simulink model "Roll_Autopilot"  (R2017b)
settings: Solver=VariableStepAuto  StartTime=0.0  StopTime=10.0  RelTol=1e-3
model workspace (MAT data in the model file):
  ContractValidatorBlocksMap = containers.Map
  ContractValidatorBlocksMap.serialization.keys = {'Roll_Autopilot/Roll_Autopilot_RollAutopilotSpec/validator', 'Roll_Autopilot/Roll_Autopilot_RollAutopilotSpec1/validator'}
  ContractValidatorBlocksMap.serialization.values{1}.block = 'Roll_Autopilot/Roll_Autopilot_RollAutopilotSpec/validator'
  ContractValidatorBlocksMap.serialization.values{1}.assumePorts = 0
  ContractValidatorBlocksMap.serialization.values{1}.guaranteePorts = 6
  ContractValidatorBlocksMap.serialization.values{1}.modeBlocksPorts = 2
  ContractValidatorBlocksMap.serialization.values{1}.portHandles.Inport = [3068.00048828 3069.00048828 3070.00048828 3071.00048828 3072.00231934 3074.00231934 3078.00231934 3079.00231934]
  ContractValidatorBlocksMap.serialization.values{1}.portHandles.Outport = 3080.00231934
  ContractValidatorBlocksMap.serialization.values{1}.portHandles.Enable = []
  ContractValidatorBlocksMap.serialization.values{1}.portHandles.Trigger = []
  ContractValidatorBlocksMap.serialization.values{1}.portHandles.State = []
  ContractValidatorBlocksMap.serialization.values{1}.portHandles.LConn = []
  ContractValidatorBlocksMap.serialization.values{1}.portHandles.RConn = []
  ContractValidatorBlocksMap.serialization.values{1}.portHandles.Ifaction = []
  ContractValidatorBlocksMap.serialization.values{1}.portHandles.Reset = []
  ContractValidatorBlocksMap.serialization.values{1}.portConnectivity(1).Type = '1'
  ContractValidatorBlocksMap.serialization.values{1}.portConnectivity(1).Position = [31840 -150]
  ContractValidatorBlocksMap.serialization.values{1}.portConnectivity(1).SrcBlock = 1525.00219727
  ContractValidatorBlocksMap.serialization.values{1}.portConnectivity(1).SrcPort = 0
  ContractValidatorBlocksMap.serialization.values{1}.portConnectivity(1).DstBlock = []
  ContractValidatorBlocksMap.serialization.values{1}.portConnectivity(1).DstPort = []
  ContractValidatorBlocksMap.serialization.values{1}.portConnectivity(2).Type = '2'
  ContractValidatorBlocksMap.serialization.values{1}.portConnectivity(2).Position = [31840 -85]
  ContractValidatorBlocksMap.serialization.values{1}.portConnectivity(2).SrcBlock = 1545.00048828
  ContractValidatorBlocksMap.serialization.values{1}.portConnectivity(2).SrcPort = 0
  ContractValidatorBlocksMap.serialization.values{1}.portConnectivity(2).DstBlock = []
  ContractValidatorBlocksMap.serialization.values{1}.portConnectivity(2).DstPort = []
  ContractValidatorBlocksMap.serialization.values{1}.portConnectivity(3).Type = '3'
  ContractValidatorBlocksMap.serialization.values{1}.portConnectivity(3).Position = [31840 -20]
  ContractValidatorBlocksMap.serialization.values{1}.portConnectivity(3).SrcBlock = 1541.00048828
  ContractValidatorBlocksMap.serialization.values{1}.portConnectivity(3).SrcPort = 0
  ContractValidatorBlocksMap.serialization.values{1}.portConnectivity(3).DstBlock = []
  ContractValidatorBlocksMap.serialization.values{1}.portConnectivity(3).DstPort = []
  ContractValidatorBlocksMap.serialization.values{1}.portConnectivity(4).Type = '4'
  ContractValidatorBlocksMap.serialization.values{1}.portConnectivity(4).Position = [31840 45]
  ContractValidatorBlocksMap.serialization.values{1}.portConnectivity(4).SrcBlock = 1537.00048828
  ContractValidatorBlocksMap.serialization.values{1}.portConnectivity(4).SrcPort = 0
  ContractValidatorBlocksMap.serialization.values{1}.portConnectivity(4).DstBlock = []
  ContractValidatorBlocksMap.serialization.values{1}.portConnectivity(4).DstPort = []
  ContractValidatorBlocksMap.serialization.values{1}.portConnectivity(5).Type = '5'
  ContractValidatorBlocksMap.serialization.values{1}.portConnectivity(5).Position = [31840 110]
  ContractValidatorBlocksMap.serialization.values{1}.portConnectivity(5).SrcBlock = 1533.00219727
  ContractValidatorBlocksMap.serialization.values{1}.portConnectivity(5).SrcPort = 0
  ContractValidatorBlocksMap.serialization.values{1}.portConnectivity(5).DstBlock = []
  ContractValidatorBlocksMap.serialization.values{1}.portConnectivity(5).DstPort = []
  ContractValidatorBlocksMap.serialization.values{1}.portConnectivity(6).Type = '6'
  ContractValidatorBlocksMap.serialization.values{1}.portConnectivity(6).Position = [31840 175]
  ContractValidatorBlocksMap.serialization.values{1}.portConnectivity(6).SrcBlock = 1549.00048828
  ContractValidatorBlocksMap.serialization.values{1}.portConnectivity(6).SrcPort = 0
  ContractValidatorBlocksMap.serialization.values{1}.portConnectivity(6).DstBlock = []
  ContractValidatorBlocksMap.serialization.values{1}.portConnectivity(6).DstPort = []
  ContractValidatorBlocksMap.serialization.values{1}.portConnectivity(7).Type = '7'
  ContractValidatorBlocksMap.serialization.values{1}.portConnectivity(7).Position = [31840 240]
  ContractValidatorBlocksMap.serialization.values{1}.portConnectivity(7).SrcBlock = 2047.00048828
  ContractValidatorBlocksMap.serialization.values{1}.portConnectivity(7).SrcPort = 0
  ContractValidatorBlocksMap.serialization.values{1}.portConnectivity(7).DstBlock = []
  ContractValidatorBlocksMap.serialization.values{1}.portConnectivity(7).DstPort = []
  ContractValidatorBlocksMap.serialization.values{1}.portConnectivity(8).Type = '8'
  ContractValidatorBlocksMap.serialization.values{1}.portConnectivity(8).Position = [31840 305]
  ContractValidatorBlocksMap.serialization.values{1}.portConnectivity(8).SrcBlock = 2007.00048828
  ContractValidatorBlocksMap.serialization.values{1}.portConnectivity(8).SrcPort = 0
  ContractValidatorBlocksMap.serialization.values{1}.portConnectivity(8).DstBlock = []
  ContractValidatorBlocksMap.serialization.values{1}.portConnectivity(8).DstPort = []
  ContractValidatorBlocksMap.serialization.values{1}.portConnectivity(9).Type = '1'
  ContractValidatorBlocksMap.serialization.values{1}.portConnectivity(9).Position = [31975 80]
  ContractValidatorBlocksMap.serialization.values{1}.portConnectivity(9).SrcBlock = []
  ContractValidatorBlocksMap.serialization.values{1}.portConnectivity(9).SrcPort = []
  ContractValidatorBlocksMap.serialization.values{1}.portConnectivity(9).DstBlock = 2349.00292969
  ContractValidatorBlocksMap.serialization.values{1}.portConnectivity(9).DstPort = 0
  ContractValidatorBlocksMap.serialization.values{2}.block = 'Roll_Autopilot/Roll_Autopilot_RollAutopilotSpec1/validator'
  ContractValidatorBlocksMap.serialization.values{2}.assumePorts = 0
  ContractValidatorBlocksMap.serialization.values{2}.guaranteePorts = 6
  ContractValidatorBlocksMap.serialization.values{2}.modeBlocksPorts = 2
  ContractValidatorBlocksMap.serialization.values{2}.portHandles.Inport = [7302.00048828 7304.00048828 7306.00048828 7308.00048828 7313.00048828 7319.00048828 7322.00048828 7326.00048828]
  ContractValidatorBlocksMap.serialization.values{2}.portHandles.Outport = 7710.00048828
  ContractValidatorBlocksMap.serialization.values{2}.portHandles.Enable = []
  ContractValidatorBlocksMap.serialization.values{2}.portHandles.Trigger = []
  ContractValidatorBlocksMap.serialization.values{2}.portHandles.State = []
  ContractValidatorBlocksMap.serialization.values{2}.portHandles.LConn = []
  ContractValidatorBlocksMap.serialization.values{2}.portHandles.RConn = []
  ContractValidatorBlocksMap.serialization.values{2}.portHandles.Ifaction = []
  ContractValidatorBlocksMap.serialization.values{2}.portHandles.Reset = []
  ContractValidatorBlocksMap.serialization.values{2}.portConnectivity(1).Type = '1'
  ContractValidatorBlocksMap.serialization.values{2}.portConnectivity(1).Position = [74140 -150]
  ContractValidatorBlocksMap.serialization.values{2}.portConnectivity(1).SrcBlock = 3094.00231934
  ContractValidatorBlocksMap.serialization.values{2}.portConnectivity(1).SrcPort = 0
  ContractValidatorBlocksMap.serialization.values{2}.portConnectivity(1).DstBlock = []
  ContractValidatorBlocksMap.serialization.values{2}.portConnectivity(1).DstPort = []
  ContractValidatorBlocksMap.serialization.values{2}.portConnectivity(2).Type = '2'
  ContractValidatorBlocksMap.serialization.values{2}.portConnectivity(2).Position = [74140 -85]
  ContractValidatorBlocksMap.serialization.values{2}.portConnectivity(2).SrcBlock = 3118.00231934
  ContractValidatorBlocksMap.serialization.values{2}.portConnectivity(2).SrcPort = 0
  ContractValidatorBlocksMap.serialization.values{2}.portConnectivity(2).DstBlock = []
  ContractValidatorBlocksMap.serialization.values{2}.portConnectivity(2).DstPort = []
  ContractValidatorBlocksMap.serialization.values{2}.portConnectivity(3).Type = '3'
  ContractValidatorBlocksMap.serialization.values{2}.portConnectivity(3).Position = [74140 -20]
  ContractValidatorBlocksMap.serialization.values{2}.portConnectivity(3).SrcBlock = 3110.00231934
  ContractValidatorBlocksMap.serialization.values{2}.portConnectivity(3).SrcPort = 0
  ContractValidatorBlocksMap.serialization.values{2}.portConnectivity(3).DstBlock = []
  ContractValidatorBlocksMap.serialization.values{2}.portConnectivity(3).DstPort = []
  ContractValidatorBlocksMap.serialization.values{2}.portConnectivity(4).Type = '4'
  ContractValidatorBlocksMap.serialization.values{2}.portConnectivity(4).Position = [74140 45]
  ContractValidatorBlocksMap.serialization.values{2}.portConnectivity(4).SrcBlock = 3106.00231934
  ContractValidatorBlocksMap.serialization.values{2}.portConnectivity(4).SrcPort = 0
  ContractValidatorBlocksMap.serialization.values{2}.portConnectivity(4).DstBlock = []
  ContractValidatorBlocksMap.serialization.values{2}.portConnectivity(4).DstPort = []
  ContractValidatorBlocksMap.serialization.values{2}.portConnectivity(5).Type = '5'
  ContractValidatorBlocksMap.serialization.values{2}.portConnectivity(5).Position = [74140 110]
  ContractValidatorBlocksMap.serialization.values{2}.portConnectivity(5).SrcBlock = 3098.00231934
  ContractValidatorBlocksMap.serialization.values{2}.portConnectivity(5).SrcPort = 0
  ContractValidatorBlocksMap.serialization.values{2}.portConnectivity(5).DstBlock = []
  ContractValidatorBlocksMap.serialization.values{2}.portConnectivity(5).DstPort = []
  ContractValidatorBlocksMap.serialization.values{2}.portConnectivity(6).Type = '6'
  ContractValidatorBlocksMap.serialization.values{2}.portConnectivity(6).Position = [74140 175]
  ContractValidatorBlocksMap.serialization.values{2}.portConnectivity(6).SrcBlock = 3122.00231934
  ContractValidatorBlocksMap.serialization.values{2}.portConnectivity(6).SrcPort = 0
  ContractValidatorBlocksMap.serialization.values{2}.portConnectivity(6).DstBlock = []
  ContractValidatorBlocksMap.serialization.values{2}.portConnectivity(6).DstPort = []
  ContractValidatorBlocksMap.serialization.values{2}.portConnectivity(7).Type = '7'
  ContractValidatorBlocksMap.serialization.values{2}.portConnectivity(7).Position = [74140 240]
  ContractValidatorBlocksMap.serialization.values{2}.portConnectivity(7).SrcBlock = 3628.00061035
  ContractValidatorBlocksMap.serialization.values{2}.portConnectivity(7).SrcPort = 0
  ContractValidatorBlocksMap.serialization.values{2}.portConnectivity(7).DstBlock = []
  ContractValidatorBlocksMap.serialization.values{2}.portConnectivity(7).DstPort = []
  ContractValidatorBlocksMap.serialization.values{2}.portConnectivity(8).Type = '8'
  ContractValidatorBlocksMap.serialization.values{2}.portConnectivity(8).Position = [74140 305]
  ContractValidatorBlocksMap.serialization.values{2}.portConnectivity(8).SrcBlock = 3594.00061035
  ContractValidatorBlocksMap.serialization.values{2}.portConnectivity(8).SrcPort = 0
  ContractValidatorBlocksMap.serialization.values{2}.portConnectivity(8).DstBlock = []
  ContractValidatorBlocksMap.serialization.values{2}.portConnectivity(8).DstPort = []
  ContractValidatorBlocksMap.serialization.values{2}.portConnectivity(9).Type = '1'
  ContractValidatorBlocksMap.serialization.values{2}.portConnectivity(9).Position = [74275 80]
  ContractValidatorBlocksMap.serialization.values{2}.portConnectivity(9).SrcBlock = []
  ContractValidatorBlocksMap.serialization.values{2}.portConnectivity(9).SrcPort = []
  ContractValidatorBlocksMap.serialization.values{2}.portConnectivity(9).DstBlock = 4161.00061035
  ContractValidatorBlocksMap.serialization.values{2}.portConnectivity(9).DstPort = 0
  ContractValidatorBlocksMap.serialization.uniformity = 0
  ContractValidatorBlocksMap.serialization.keyType = 'char'
  ContractValidatorBlocksMap.serialization.valueType = 'any'
undefined symbols (not defined in the file): contractAfterSimulation, contractBeforeSimulation, ContractBlock, ContractEnsureBlock, ContractGuaranteeBlock, ContractModeBlock, ContractRequireBlock, ContractValidatorBlock, saveValidatorParameters, Ts
libraries: cocosimLibs x20, simulink x2
(part 1 of 2)
settings Model: Creator=hbourbou  LastModifiedBy=hbourbou
settings DataIOCC: ReturnWorkspaceOutputs=on
settings SFSimCC: SimUseLocalCustomCode=on
settings RTWCC: RTWUseLocalCustomCode=on

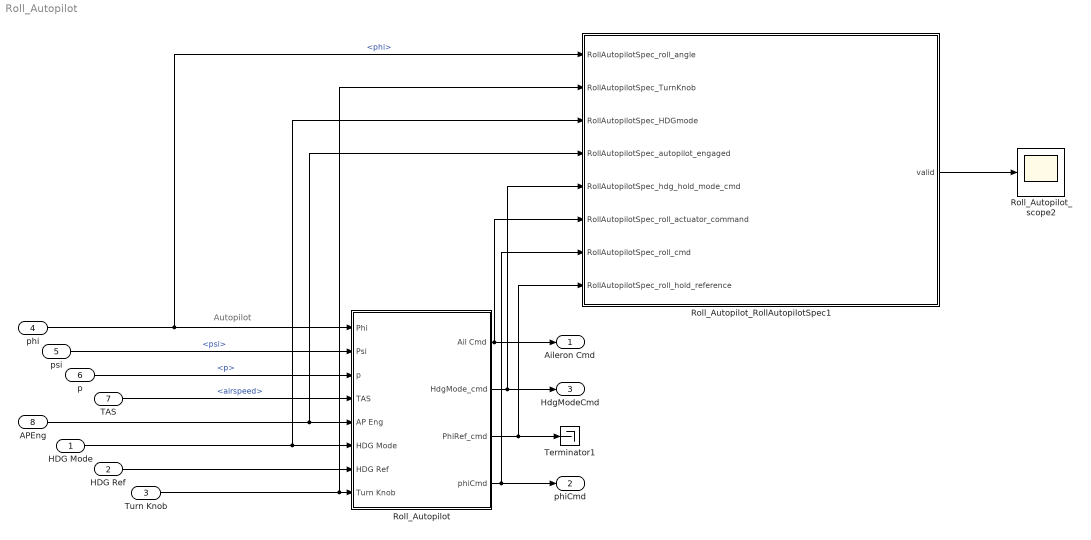
== system Roll_Autopilot ==
  note: Autopilot
  HDG Mode : Inport  OutMin=0  OutMax=1  OutDataTypeStr=boolean  PortDimensions=1
  HDG Ref : Inport  Port=2  OutMin=-180  OutMax=180  OutDataTypeStr=double  PortDimensions=1
  Turn Knob : Inport  Port=3  OutMin=-45  OutMax=45  OutDataTypeStr=double  PortDimensions=1
  phi : Inport  Port=4
  psi : Inport  Port=5
  p : Inport  Port=6
  TAS : Inport  Port=7
  APEng : Inport  Port=8  OutDataTypeStr=boolean
  Roll_Autopilot : Subsystem
  Roll_Autopilot_RollAutopilotSpec1 : Subsystem  mask(ContractBlock){ContractBlockType=ContractBlock}
      mask init:
      | set_param(gcb, 'LinkStatus', 'none');
      mask DialogControl DescTextVar Prompt: Contract block
      mask Display:
      | text(0.5, 0.5, '{\bf\fontsize{20}Contract}', 'hor', 'center', 'texmode','on');
      | blocks = find_system(gcb, 'LookUnderMasks','all', 'SearchDepth',1,'BlockType','Inport');
      | for i = 1 : length(blocks)
      |     blockName = get_param(blocks(i), 'Name');
      |     [path, blockName] = fileparts(char(blockName));
      |     port_label('input', i, blockName);
      | end
      | 
      | blocks = find_system(gcb, 'LookUnderMasks','all', 'SearchDepth',1,'BlockType','Outport');
      | for i = 1 : length(blocks)
      |     blockName = get_param(blocks(i), 'Name');
      |     [path, blockName] = fileparts(char(blockName));
      |     port_label('output', i, blockName);
      | end
  Roll_Autopilot_scope2 : Scope
  Terminator1 : Terminator
  Aileron Cmd : Outport  OutDataTypeStr=double  PortDimensions=1  SampleTime=[0.025000000000000001,0]  VectorParamsAs1DForOutWhenUnconnected=off
  phiCmd : Outport  Port=2  VectorParamsAs1DForOutWhenUnconnected=off
  HdgModeCmd : Outport  Port=3  VectorParamsAs1DForOutWhenUnconnected=off
  wires:
  APEng/1 -> Roll_Autopilot_RollAutopilotSpec1/4(RollAutopilotSpec_autopilot_engaged), Roll_Autopilot/5(AP Eng)
  TAS/1 -> Roll_Autopilot/4(TAS)  "<airspeed>"
  Roll_Autopilot/2(HdgMode_cmd) -> Roll_Autopilot_RollAutopilotSpec1/5(RollAutopilotSpec_hdg_hold_mode_cmd), HdgModeCmd/1
  Turn Knob/1 -> Roll_Autopilot_RollAutopilotSpec1/2(RollAutopilotSpec_TurnKnob), Roll_Autopilot/8(Turn Knob)
  phi/1 -> Roll_Autopilot_RollAutopilotSpec1/1(RollAutopilotSpec_roll_angle), Roll_Autopilot/1(Phi)  "<phi>"
  HDG Mode/1 -> Roll_Autopilot_RollAutopilotSpec1/3(RollAutopilotSpec_HDGmode), Roll_Autopilot/6(HDG Mode)
  HDG Ref/1 -> Roll_Autopilot/7(HDG Ref)
  p/1 -> Roll_Autopilot/3(p)  "<p>"
  Roll_Autopilot/1(Ail Cmd) -> Roll_Autopilot_RollAutopilotSpec1/6(RollAutopilotSpec_roll_actuator_command), Aileron Cmd/1
  psi/1 -> Roll_Autopilot/2(Psi)  "<psi>"
  Roll_Autopilot/4(phiCmd) -> Roll_Autopilot_RollAutopilotSpec1/7(RollAutopilotSpec_roll_cmd), phiCmd/1
  Roll_Autopilot/3(PhiRef_cmd) -> Roll_Autopilot_RollAutopilotSpec1/8(RollAutopilotSpec_roll_hold_reference), Terminator1/1
  Roll_Autopilot_RollAutopilotSpec1/1(valid) -> Roll_Autopilot_scope2/1

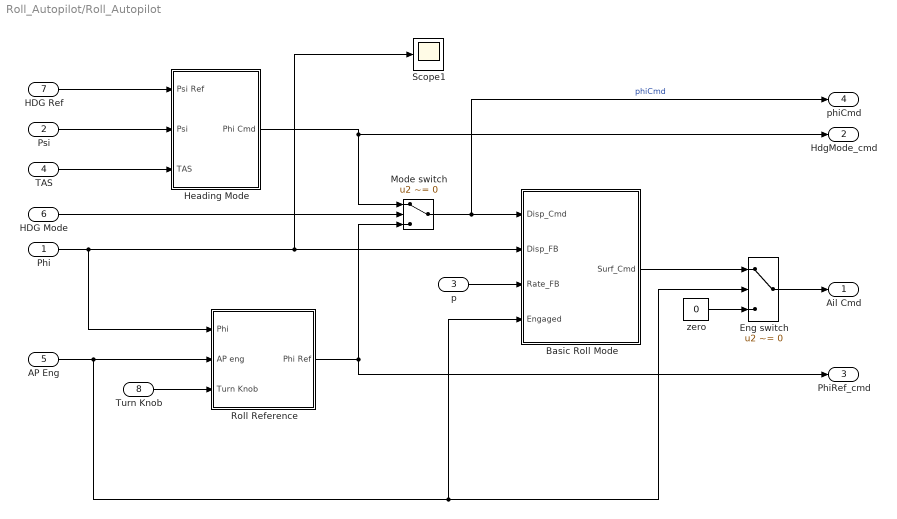
== system Roll_Autopilot/Roll_Autopilot ==
  Phi : Inport  OutMin=-180  OutMax=180  OutDataTypeStr=double  PortDimensions=1  SampleTime=1/40  Interpolate=off
  Psi : Inport  Port=2  OutMin=-180  OutMax=180  OutDataTypeStr=double  PortDimensions=1  SampleTime=1/40  Interpolate=off
  p : Inport  Port=3  OutMin=-180  OutMax=180  OutDataTypeStr=double  PortDimensions=1  Interpolate=off
  TAS : Inport  Port=4  OutMin=0  OutMax=1000  OutDataTypeStr=double  PortDimensions=1  SampleTime=1/40  Interpolate=off
  AP Eng : Inport  Port=5  OutDataTypeStr=boolean  PortDimensions=1  SampleTime=1/40  Interpolate=off
  HDG Mode : Inport  Port=6  OutDataTypeStr=boolean  PortDimensions=1  SampleTime=1/40  Interpolate=off
  HDG Ref : Inport  Port=7  OutMin=-180  OutMax=180  OutDataTypeStr=double  PortDimensions=1  SampleTime=1/40  Interpolate=off
  Turn Knob : Inport  Port=8  OutMin=-45  OutMax=45  OutDataTypeStr=double  PortDimensions=1  SampleTime=1/40  Interpolate=off
  Basic Roll Mode : Subsystem
  Eng switch : Switch  Criteria=u2 ~= 0
  Heading Mode : Subsystem
  Mode switch : Switch  Criteria=u2 ~= 0
  Roll Reference : Subsystem  TreatAsAtomicUnit=on
      settings: RTWSystemCode=Inline
  Scope1 : Scope
  zero : Constant  Value=0  OutDataTypeStr=double
  Ail Cmd : Outport  OutDataTypeStr=double  PortDimensions=1  SampleTime=1/40  VectorParamsAs1DForOutWhenUnconnected=off
  HdgMode_cmd : Outport  Port=2  VectorParamsAs1DForOutWhenUnconnected=off
  PhiRef_cmd : Outport  Port=3  VectorParamsAs1DForOutWhenUnconnected=off
  phiCmd : Outport  Port=4  VectorParamsAs1DForOutWhenUnconnected=off
  wires:
  HDG Ref/1 -> Heading Mode/1(Psi Ref)
  Heading Mode/1(Phi Cmd) -> HdgMode_cmd/1, Mode switch/1
  Mode switch/1 -> phiCmd/1, Basic Roll Mode/1(Disp_Cmd)  "phiCmd"
  Eng switch/1 -> Ail Cmd/1
  AP Eng/1 -> Roll Reference/2(AP eng), Basic Roll Mode/4(Engaged), Eng switch/2
  TAS/1 -> Heading Mode/3(TAS)
  HDG Mode/1 -> Mode switch/2
  Roll Reference/1(Phi Ref) -> Mode switch/3, PhiRef_cmd/1
  Turn Knob/1 -> Roll Reference/3(Turn Knob)
  zero/1 -> Eng switch/3
  p/1 -> Basic Roll Mode/3(Rate_FB)
  Phi/1 -> Scope1/1, Basic Roll Mode/2("Disp_FB "), Roll Reference/1(Phi)
  Psi/1 -> Heading Mode/2(Psi)
  Basic Roll Mode/1(Surf_Cmd) -> Eng switch/1

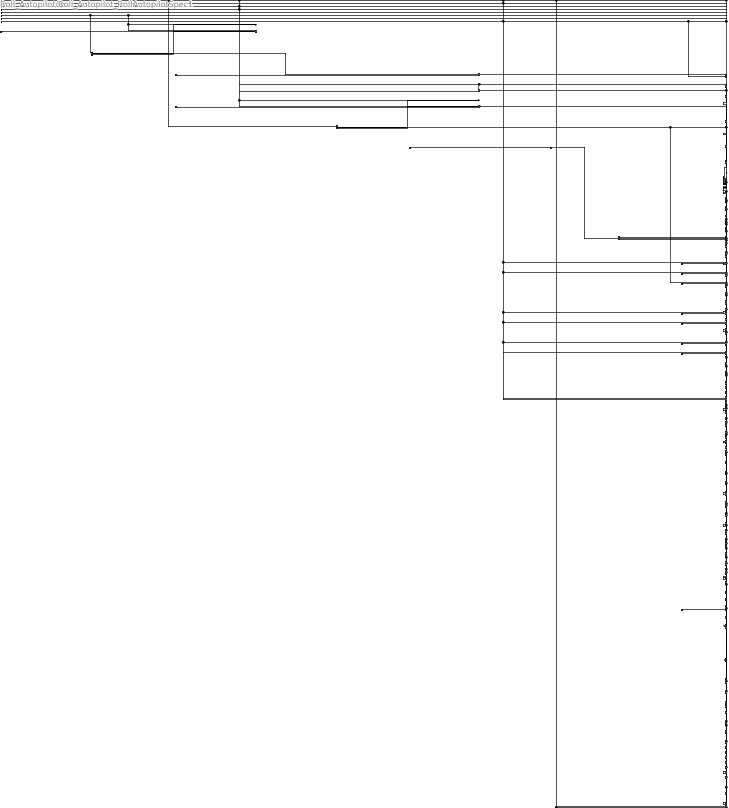
== system Roll_Autopilot/Roll_Autopilot_RollAutopilotSpec1 ==
  RollAutopilotSpec_roll_angle : Inport  OutDataTypeStr=double
  RollAutopilotSpec_TurnKnob : Inport  Port=2  OutDataTypeStr=double
  RollAutopilotSpec_HDGmode : Inport  Port=3  OutDataTypeStr=boolean
  RollAutopilotSpec_autopilot_engaged : Inport  Port=4  OutDataTypeStr=boolean
  RollAutopilotSpec_hdg_hold_mode_cmd : Inport  Port=5  OutDataTypeStr=double
  RollAutopilotSpec_roll_actuator_command : Inport  Port=6  OutDataTypeStr=double
  RollAutopilotSpec_roll_cmd : Inport  Port=7  OutDataTypeStr=double
  RollAutopilotSpec_roll_hold_reference : Inport  Port=8  OutDataTypeStr=double
  AP-001 : Subsystem  mask(ContractGuaranteeBlock){ContractBlockType=ContractGuaranteeBlock}
      mask init:
      | set_param(gcb, 'LinkStatus', 'none');
      mask DialogControl DescTextVar Prompt: Guarantee block
  AP-003A : Subsystem  mask(ContractGuaranteeBlock){ContractBlockType=ContractGuaranteeBlock}
      mask init:
      | set_param(gcb, 'LinkStatus', 'none');
      mask DialogControl DescTextVar Prompt: Guarantee block
  AP-003B : Subsystem  mask(ContractGuaranteeBlock){ContractBlockType=ContractGuaranteeBlock}
      mask init:
      | set_param(gcb, 'LinkStatus', 'none');
      mask DialogControl DescTextVar Prompt: Guarantee block
  AP-003C : Subsystem  mask(ContractGuaranteeBlock){ContractBlockType=ContractGuaranteeBlock}
      mask init:
      | set_param(gcb, 'LinkStatus', 'none');
      mask DialogControl DescTextVar Prompt: Guarantee block
  AP-003D : Subsystem  mask(ContractGuaranteeBlock){ContractBlockType=ContractGuaranteeBlock}
      mask init:
      | set_param(gcb, 'LinkStatus', 'none');
      mask DialogControl DescTextVar Prompt: Guarantee block
  AP-007 : Subsystem  mask(ContractGuaranteeBlock){ContractBlockType=ContractGuaranteeBlock}
      mask init:
      | set_param(gcb, 'LinkStatus', 'none');
      mask DialogControl DescTextVar Prompt: Guarantee block
  Arrow_xxRollAutopilotSpec_162_ni_7 : Delay  DelayLength=1  InitialCondition=1
  Arrow_xxRollAutopilotSpec_163_ni_9 : Delay  DelayLength=1  InitialCondition=1
  Arrow_xxRollAutopilotSpec_164_ni_12 : Delay  DelayLength=1  InitialCondition=1
  Arrow_xxRollAutopilotSpec_165_ni_16 : Delay  DelayLength=1  InitialCondition=1
  Arrow_xxRollAutopilotSpec_183_ni_3 : Delay  DelayLength=1  InitialCondition=1
  Ca_operator : Logic  Operator=NOT  AllPortsSameDT=off  OutDataTypeStr=boolean
  Cb_operator : Logic  AllPortsSameDT=off  OutDataTypeStr=boolean
  Cc_operator : RelationalOperator  OutDataTypeStr=boolean  RndMeth=Simplest
  Cc_rhs_2 : Constant  Value=30.0  OutDataTypeStr=double
  Cd_operator : Logic  AllPortsSameDT=off  OutDataTypeStr=boolean
  H_call : Subsystem
  H_call1 : Subsystem
  H_call11 : Subsystem
  PRE_xxRollAutopilotSpec_{8,13,17,22,33,38,42,44,59,64,68,73,84,89,93,95,109,114,118,123,133,138,142,144,184,187} (26 alike) : Delay  DelayLength=1  InitialCondition=0
  SI_call : Subsystem
  SI_call1 : Subsystem
  SI_call11 : Subsystem
  SI_call111 : Subsystem
  SI_call1111 : Subsystem
  SI_call11111 : Subsystem
  SI_call111111 : Subsystem
  SI_call1111111 : Subsystem
  SI_call11111111 : Subsystem
  branch_10_IF : Switch  Criteria=u2 ~= 0
  branch_11_IF : Switch  Criteria=u2 ~= 0
  branch_12_IF : Switch  Criteria=u2 ~= 0
  branch_13_IF : Switch  Criteria=u2 ~= 0
  branch_14_IF : Switch  Criteria=u2 ~= 0
  branch_15_IF : Switch  Criteria=u2 ~= 0
  branch_16_IF : Switch  Criteria=u2 ~= 0
  branch_8_IF : Switch  Criteria=u2 ~= 0
  branch_9_IF : Switch  Criteria=u2 ~= 0
  hdg_hold_mode : Subsystem  mask(ContractModeBlock){ContractBlockType=ContractModeBlock}
      mask init:
      | set_param(gcb, 'LinkStatus', 'none');
      mask DialogControl DescTextVar Prompt: Mode block
  hdg_hold_mode_ensure : Subsystem  mask(ContractEnsureBlock){ContractBlockType=ContractEnsureBlock}
      mask init:
      | set_param(gcb, 'LinkStatus', 'none');
      mask DialogControl DescTextVar Prompt: Ensure block
  hdg_hold_mode_ensure_cond : Logic  Inputs=1  AllPortsSameDT=off  OutDataTypeStr=boolean
  hdg_hold_mode_require : Subsystem  mask(ContractRequireBlock){ContractBlockType=ContractRequireBlock}
      mask init:
      | set_param(gcb, 'LinkStatus', 'none');
      mask DialogControl DescTextVar Prompt: Require block
  hdg_hold_mode_require_cond : Logic  Inputs=1  AllPortsSameDT=off  OutDataTypeStr=boolean
  no_other_lateral_mode_operator : Logic  Operator=NOT  AllPortsSameDT=off  OutDataTypeStr=boolean
  roll_hold_mode : Subsystem  mask(ContractModeBlock){ContractBlockType=ContractModeBlock}
      mask init:
      | set_param(gcb, 'LinkStatus', 'none');
      mask DialogControl DescTextVar Prompt: Mode block
  roll_hold_mode_ensure : Subsystem  mask(ContractEnsureBlock){ContractBlockType=ContractEnsureBlock}
      mask init:
      | set_param(gcb, 'LinkStatus', 'none');
      mask DialogControl DescTextVar Prompt: Ensure block
  roll_hold_mode_ensure_cond : Logic  Inputs=1  AllPortsSameDT=off  OutDataTypeStr=boolean
  roll_hold_mode_require : Subsystem  mask(ContractRequireBlock){ContractBlockType=ContractRequireBlock}
      mask init:
      | set_param(gcb, 'LinkStatus', 'none');
      mask DialogControl DescTextVar Prompt: Require block
  roll_hold_mode_require_cond : Logic  Inputs=1  AllPortsSameDT=off  OutDataTypeStr=boolean
  roll_hold_operator : Logic  AllPortsSameDT=off  OutDataTypeStr=boolean
  spec206_operator : cocosimLibs/Implies  SystemSampleTime=-1  Latency=0  AutoFrameSizeCalculation=off
  spec211_operator : Logic  AllPortsSameDT=off  OutDataTypeStr=boolean
  spec216_operator : RelationalOperator  Operator===  OutDataTypeStr=boolean  RndMeth=Simplest
  spec223_operator : RelationalOperator  Operator===  OutDataTypeStr=boolean  RndMeth=Simplest
  spec252_operator : cocosimLibs/Implies  SystemSampleTime=-1  Latency=0  AutoFrameSizeCalculation=off
  spec621_operator : RelationalOperator  Operator=<=  OutDataTypeStr=boolean  RndMeth=Simplest
  spec621_rhs_2 : Constant  Value=15.0  OutDataTypeStr=double
  validator : M-S-Function  LoadFcn=saveValidatorParameters(gcb);  InitFcn=contractBeforeSimulation();  StopFcn=contractAfterSimulation();  FunctionName=contract  mask(ContractValidatorBlock){assumePorts=0, guaranteePorts=6, modePorts=2, ContractBlockType=ContractValidatorBlock, createInportsCheckbox=off}
      mask prompts: assumePorts "Assume ports     :"; guaranteePorts "Guarantee ports :"; modePorts "Mode ports        :"; createInportsCheckbox "Create inports and connect them automatically"
      mask init:
      | set_param(gcb,'LinkStatus','none');
      | contract_callback('inputs_callback',gcb);
      mask DialogControl DescTextVar Prompt: The validator block implements the following logic: <br> <br> <b>Sofar</b>(assume<sub>1</sub> <b>&#8743;</b> assume<sub>2</sub> <b>&#8743;</b> ... assume<sub>k</sub>) <b>&rarr;</b> (guarantee<sub>1</sub> <b>&#8743;</b> guarantee<sub>2</sub> <b>&#8743;</b> ... guarantee<sub>m</sub> <b>&#8743;</b>  mode<sub>1</sub> <b>&#8743;</b> mode<sub>2</sub> <b>&#8743;</b> ... <b>&#8743;</b> mode<sub>n</sub> )<br> where mode<sub>i</sub> = require<sub>i</sub> <b>&rarr;</b> ensure<sub>i</sub>
      mask Display:
      | color('black');
      | port_label('input',1,'guarantee');
      | port_label('input',2,'guarantee');
      | port_label('input',3,'guarantee');
      | port_label('input',4,'guarantee');
      | port_label('input',5,'guarantee');
      | port_label('input',6,'guarantee');
      | port_label('input',7,'mode');
      | port_label('input',8,'mode');
      | port_label('output',1,'valid');
  xxRollAutopilotSpec_101_operator : Logic  AllPortsSameDT=off  OutDataTypeStr=boolean
  xxRollAutopilotSpec_102_rhs1 : Constant  Value=true  OutDataTypeStr=boolean
  xxRollAutopilotSpec_104_operator : Product  OutDataTypeStr=double
  xxRollAutopilotSpec_104_rhs_1 : Constant  Value=30.0  OutDataTypeStr=double
  xxRollAutopilotSpec_105_operator : RelationalOperator  Operator===  OutDataTypeStr=boolean  RndMeth=Simplest
  xxRollAutopilotSpec_106_operator : RelationalOperator  OutDataTypeStr=boolean  RndMeth=Simplest
  xxRollAutopilotSpec_106_rhs_2 : Constant  Value=30.0  OutDataTypeStr=double
  xxRollAutopilotSpec_107_operator : cocosimLibs/Implies  SystemSampleTime=-1  Latency=0  AutoFrameSizeCalculation=off
  xxRollAutopilotSpec_108_operator : Logic  Operator=NOT  AllPortsSameDT=off  OutDataTypeStr=boolean
  xxRollAutopilotSpec_10_operator : Logic  AllPortsSameDT=off  OutDataTypeStr=boolean
  xxRollAutopilotSpec_110_operator : Logic  Operator=OR  AllPortsSameDT=off  OutDataTypeStr=boolean
  xxRollAutopilotSpec_111_operator : Logic  AllPortsSameDT=off  OutDataTypeStr=boolean
  xxRollAutopilotSpec_112_operator : cocosimLibs/Implies  SystemSampleTime=-1  Latency=0  AutoFrameSizeCalculation=off
  xxRollAutopilotSpec_113_operator : Logic  Operator=NOT  AllPortsSameDT=off  OutDataTypeStr=boolean
  xxRollAutopilotSpec_115_operator : Logic  Operator=OR  AllPortsSameDT=off  OutDataTypeStr=boolean
  xxRollAutopilotSpec_116_operator : Logic  AllPortsSameDT=off  OutDataTypeStr=boolean
  xxRollAutopilotSpec_119_operator : Logic  Operator=NOT  AllPortsSameDT=off  OutDataTypeStr=boolean
  xxRollAutopilotSpec_11_operator : cocosimLibs/Implies  SystemSampleTime=-1  Latency=0  AutoFrameSizeCalculation=off
  xxRollAutopilotSpec_120_operator : Logic  AllPortsSameDT=off  OutDataTypeStr=boolean
  xxRollAutopilotSpec_121_operator : Logic  Operator=NOT  AllPortsSameDT=off  OutDataTypeStr=boolean
  xxRollAutopilotSpec_122_operator : Logic  Operator=NOT  AllPortsSameDT=off  OutDataTypeStr=boolean
  xxRollAutopilotSpec_124_operator : Logic  Operator=OR  AllPortsSameDT=off  OutDataTypeStr=boolean
  xxRollAutopilotSpec_125_operator : Logic  AllPortsSameDT=off  OutDataTypeStr=boolean
  xxRollAutopilotSpec_127_operator : cocosimLibs/Implies  SystemSampleTime=-1  Latency=0  AutoFrameSizeCalculation=off
  xxRollAutopilotSpec_128_operator : Product  OutDataTypeStr=double
  xxRollAutopilotSpec_128_rhs_1 : Constant  Value=30.0  OutDataTypeStr=double
  xxRollAutopilotSpec_129_operator : RelationalOperator  Operator===  OutDataTypeStr=boolean  RndMeth=Simplest
  xxRollAutopilotSpec_12_operator : Logic  Operator=NOT  AllPortsSameDT=off  OutDataTypeStr=boolean
  xxRollAutopilotSpec_130_operator : RelationalOperator  OutDataTypeStr=boolean  RndMeth=Simplest
  xxRollAutopilotSpec_130_rhs_2 : Constant  Value=30.0  OutDataTypeStr=double
  xxRollAutopilotSpec_131_operator : cocosimLibs/Implies  SystemSampleTime=-1  Latency=0  AutoFrameSizeCalculation=off
  xxRollAutopilotSpec_132_operator : Logic  Operator=NOT  AllPortsSameDT=off  OutDataTypeStr=boolean
  xxRollAutopilotSpec_134_operator : Logic  Operator=OR  AllPortsSameDT=off  OutDataTypeStr=boolean
  xxRollAutopilotSpec_135_operator : Logic  AllPortsSameDT=off  OutDataTypeStr=boolean
  xxRollAutopilotSpec_136_operator : cocosimLibs/Implies  SystemSampleTime=-1  Latency=0  AutoFrameSizeCalculation=off
  xxRollAutopilotSpec_137_operator : Logic  Operator=NOT  AllPortsSameDT=off  OutDataTypeStr=boolean
  xxRollAutopilotSpec_139_operator : Logic  Operator=OR  AllPortsSameDT=off  OutDataTypeStr=boolean
  xxRollAutopilotSpec_140_operator : Logic  AllPortsSameDT=off  OutDataTypeStr=boolean
  xxRollAutopilotSpec_143_operator : Logic  Operator=NOT  AllPortsSameDT=off  OutDataTypeStr=boolean
  xxRollAutopilotSpec_145_operator : Logic  Operator=NOT  AllPortsSameDT=off  OutDataTypeStr=boolean
  xxRollAutopilotSpec_146_operator : Logic  AllPortsSameDT=off  OutDataTypeStr=boolean
  xxRollAutopilotSpec_147_operator : Logic  AllPortsSameDT=off  OutDataTypeStr=boolean
  xxRollAutopilotSpec_148_operator : cocosimLibs/Implies  SystemSampleTime=-1  Latency=0  AutoFrameSizeCalculation=off
  xxRollAutopilotSpec_14_operator : Logic  Operator=OR  AllPortsSameDT=off  OutDataTypeStr=boolean
  xxRollAutopilotSpec_150_operator : Logic  AllPortsSameDT=off  OutDataTypeStr=boolean
  xxRollAutopilotSpec_151_rhs1 : Constant  Value=true  OutDataTypeStr=boolean
  xxRollAutopilotSpec_152_operator : RelationalOperator  Operator===  OutDataTypeStr=boolean  RndMeth=Simplest
  xxRollAutopilotSpec_153_operator : RelationalOperator  OutDataTypeStr=boolean  RndMeth=Simplest
  xxRollAutopilotSpec_153_rhs_2 : Constant  Value=-30.0  OutDataTypeStr=double
  xxRollAutopilotSpec_154_operator : RelationalOperator  Operator=<=  OutDataTypeStr=boolean  RndMeth=Simplest
  xxRollAutopilotSpec_154_rhs_2 : Constant  Value=30.0  OutDataTypeStr=double
  xxRollAutopilotSpec_155_operator : Logic  Operator=OR  AllPortsSameDT=off  OutDataTypeStr=boolean
  xxRollAutopilotSpec_156_operator : RelationalOperator  Operator=<=  OutDataTypeStr=boolean  RndMeth=Simplest
  xxRollAutopilotSpec_156_rhs_2 : Constant  Value=-3.0  OutDataTypeStr=double
  xxRollAutopilotSpec_157_operator : RelationalOperator  OutDataTypeStr=boolean  RndMeth=Simplest
  xxRollAutopilotSpec_157_rhs_2 : Constant  Value=3.0  OutDataTypeStr=double
  xxRollAutopilotSpec_158_operator : Logic  Operator=OR  AllPortsSameDT=off  OutDataTypeStr=boolean
  xxRollAutopilotSpec_159_operator : Logic  AllPortsSameDT=off  OutDataTypeStr=boolean
  xxRollAutopilotSpec_15_operator : Logic  AllPortsSameDT=off  OutDataTypeStr=boolean
  xxRollAutopilotSpec_160_operator : RelationalOperator  Operator===  OutDataTypeStr=boolean  RndMeth=Simplest
  xxRollAutopilotSpec_160_rhs_2 : Constant  Value=0.0  OutDataTypeStr=double
  xxRollAutopilotSpec_161_operator : Logic  Operator=NOT  AllPortsSameDT=off  OutDataTypeStr=boolean
  xxRollAutopilotSpec_162_ni_7_init : Constant  Value=0  OutDataTypeStr=boolean
  xxRollAutopilotSpec_163_ni_9_init : Constant  Value=0  OutDataTypeStr=boolean
  xxRollAutopilotSpec_164_ni_12_init : Constant  Value=0  OutDataTypeStr=boolean
  xxRollAutopilotSpec_165_ni_16_init : Constant  Value=0  OutDataTypeStr=boolean
  xxRollAutopilotSpec_166_rhs : Constant  Value=false  OutDataTypeStr=boolean
  xxRollAutopilotSpec_166_rhs1 : Constant  Value=true  OutDataTypeStr=boolean
  xxRollAutopilotSpec_167_operator : RelationalOperator  OutDataTypeStr=boolean  RndMeth=Simplest
  xxRollAutopilotSpec_167_rhs_2 : Constant  Value=0.0  OutDataTypeStr=double
  xxRollAutopilotSpec_168_operator : Gain  Gain=-1  OutDataTypeStr=double
  xxRollAutopilotSpec_169_operator : RelationalOperator  OutDataTypeStr=boolean  RndMeth=Simplest
  xxRollAutopilotSpec_169_rhs_2 : Constant  Value=0.0  OutDataTypeStr=double
  xxRollAutopilotSpec_170_operator : Gain  Gain=-1  OutDataTypeStr=double
  xxRollAutopilotSpec_171_rhs : Constant  Value=1.0  OutDataTypeStr=double
  xxRollAutopilotSpec_172_rhs : Constant  Value=-1.0  OutDataTypeStr=double
  xxRollAutopilotSpec_173_operator : RelationalOperator  Operator=<  OutDataTypeStr=boolean  RndMeth=Simplest
  xxRollAutopilotSpec_173_rhs_2 : Constant  Value=6.0  OutDataTypeStr=double
  xxRollAutopilotSpec_174_operator : RelationalOperator  Operator=>  OutDataTypeStr=boolean  RndMeth=Simplest
  xxRollAutopilotSpec_174_rhs_2 : Constant  Value=-6.0  OutDataTypeStr=double
  xxRollAutopilotSpec_175_operator : RelationalOperator  OutDataTypeStr=boolean  RndMeth=Simplest
  xxRollAutopilotSpec_175_rhs_2 : Constant  Value=-30.0  OutDataTypeStr=double
  xxRollAutopilotSpec_176_operator : RelationalOperator  Operator=<=  OutDataTypeStr=boolean  RndMeth=Simplest
  xxRollAutopilotSpec_176_rhs_2 : Constant  Value=30.0  OutDataTypeStr=double
  xxRollAutopilotSpec_177_operator : Logic  Operator=OR  AllPortsSameDT=off  OutDataTypeStr=boolean
  xxRollAutopilotSpec_178_operator : RelationalOperator  Operator=<=  OutDataTypeStr=boolean  RndMeth=Simplest
  xxRollAutopilotSpec_178_rhs_2 : Constant  Value=-3.0  OutDataTypeStr=double
  xxRollAutopilotSpec_179_operator : RelationalOperator  OutDataTypeStr=boolean  RndMeth=Simplest
  xxRollAutopilotSpec_179_rhs_2 : Constant  Value=3.0  OutDataTypeStr=double
  xxRollAutopilotSpec_180_operator : Logic  Operator=OR  AllPortsSameDT=off  OutDataTypeStr=boolean
  xxRollAutopilotSpec_181_operator : Logic  Operator=OR  AllPortsSameDT=off  OutDataTypeStr=boolean
  xxRollAutopilotSpec_182_operator : Logic  Operator=OR  AllPortsSameDT=off  OutDataTypeStr=boolean
  xxRollAutopilotSpec_183_ni_3_init : Constant  Value=0  OutDataTypeStr=boolean
  xxRollAutopilotSpec_185_rhs1 : Constant  Value=false  OutDataTypeStr=boolean
  xxRollAutopilotSpec_186_rhs : Constant  Value=0.0  OutDataTypeStr=double
  xxRollAutopilotSpec_18_operator : Logic  Operator=NOT  AllPortsSameDT=off  OutDataTypeStr=boolean
  xxRollAutopilotSpec_19_operator : Logic  AllPortsSameDT=off  OutDataTypeStr=boolean
  xxRollAutopilotSpec_20_operator : Logic  Operator=NOT  AllPortsSameDT=off  OutDataTypeStr=boolean
  xxRollAutopilotSpec_21_operator : Logic  Operator=NOT  AllPortsSameDT=off  OutDataTypeStr=boolean
  xxRollAutopilotSpec_23_operator : Logic  Operator=OR  AllPortsSameDT=off  OutDataTypeStr=boolean
  xxRollAutopilotSpec_24_operator : Logic  AllPortsSameDT=off  OutDataTypeStr=boolean
  xxRollAutopilotSpec_26_operator : cocosimLibs/Implies  SystemSampleTime=-1  Latency=0  AutoFrameSizeCalculation=off
  xxRollAutopilotSpec_27_operator : RelationalOperator  Operator===  OutDataTypeStr=boolean  RndMeth=Simplest
  xxRollAutopilotSpec_28_operator : Logic  Operator=OR  AllPortsSameDT=off  OutDataTypeStr=boolean
  xxRollAutopilotSpec_29_operator : Logic  Operator=OR  AllPortsSameDT=off  OutDataTypeStr=boolean
  xxRollAutopilotSpec_2_operator : RelationalOperator  Operator===  OutDataTypeStr=boolean  RndMeth=Simplest
  xxRollAutopilotSpec_30_operator : Logic  Operator=NOT  AllPortsSameDT=off  OutDataTypeStr=boolean
  xxRollAutopilotSpec_31_operator : cocosimLibs/Implies  SystemSampleTime=-1  Latency=0  AutoFrameSizeCalculation=off
  xxRollAutopilotSpec_32_operator : Logic  Operator=NOT  AllPortsSameDT=off  OutDataTypeStr=boolean
  xxRollAutopilotSpec_34_operator : Logic  Operator=OR  AllPortsSameDT=off  OutDataTypeStr=boolean
  xxRollAutopilotSpec_35_operator : Logic  AllPortsSameDT=off  OutDataTypeStr=boolean
  xxRollAutopilotSpec_36_operator : cocosimLibs/Implies  SystemSampleTime=-1  Latency=0  AutoFrameSizeCalculation=off
  xxRollAutopilotSpec_37_operator : Logic  Operator=NOT  AllPortsSameDT=off  OutDataTypeStr=boolean
  xxRollAutopilotSpec_39_operator : Logic  Operator=OR  AllPortsSameDT=off  OutDataTypeStr=boolean
  xxRollAutopilotSpec_3_operator : Logic  Operator=OR  AllPortsSameDT=off  OutDataTypeStr=boolean
  xxRollAutopilotSpec_40_operator : Logic  AllPortsSameDT=off  OutDataTypeStr=boolean
  xxRollAutopilotSpec_43_operator : Logic  Operator=NOT  AllPortsSameDT=off  OutDataTypeStr=boolean
  xxRollAutopilotSpec_45_operator : Logic  Operator=NOT  AllPortsSameDT=off  OutDataTypeStr=boolean
  xxRollAutopilotSpec_46_operator : Logic  AllPortsSameDT=off  OutDataTypeStr=boolean
  xxRollAutopilotSpec_47_operator : Logic  AllPortsSameDT=off  OutDataTypeStr=boolean
  xxRollAutopilotSpec_48_operator : cocosimLibs/Implies  SystemSampleTime=-1  Latency=0  AutoFrameSizeCalculation=off
  xxRollAutopilotSpec_4_operator : Logic  Operator=OR  AllPortsSameDT=off  OutDataTypeStr=boolean
  xxRollAutopilotSpec_50_operator : Logic  AllPortsSameDT=off  OutDataTypeStr=boolean
  xxRollAutopilotSpec_51_rhs1 : Constant  Value=true  OutDataTypeStr=boolean
  xxRollAutopilotSpec_53_operator : RelationalOperator  Operator===  OutDataTypeStr=boolean  RndMeth=Simplest
  xxRollAutopilotSpec_53_rhs_2 : Constant  Value=0.0  OutDataTypeStr=double
  xxRollAutopilotSpec_54_operator : RelationalOperator  Operator=>  OutDataTypeStr=boolean  RndMeth=Simplest
  xxRollAutopilotSpec_54_rhs_2 : Constant  Value=-6.0  OutDataTypeStr=double
  xxRollAutopilotSpec_55_operator : RelationalOperator  Operator=<  OutDataTypeStr=boolean  RndMeth=Simplest
  xxRollAutopilotSpec_55_rhs_2 : Constant  Value=6.0  OutDataTypeStr=double
  xxRollAutopilotSpec_56_operator : Logic  AllPortsSameDT=off  OutDataTypeStr=boolean
  xxRollAutopilotSpec_57_operator : cocosimLibs/Implies  SystemSampleTime=-1  Latency=0  AutoFrameSizeCalculation=off
  xxRollAutopilotSpec_58_operator : Logic  Operator=NOT  AllPortsSameDT=off  OutDataTypeStr=boolean
  xxRollAutopilotSpec_5_operator : Logic  Operator=NOT  AllPortsSameDT=off  OutDataTypeStr=boolean
  xxRollAutopilotSpec_60_operator : Logic  Operator=OR  AllPortsSameDT=off  OutDataTypeStr=boolean
  xxRollAutopilotSpec_61_operator : Logic  AllPortsSameDT=off  OutDataTypeStr=boolean
  xxRollAutopilotSpec_62_operator : cocosimLibs/Implies  SystemSampleTime=-1  Latency=0  AutoFrameSizeCalculation=off
  xxRollAutopilotSpec_63_operator : Logic  Operator=NOT  AllPortsSameDT=off  OutDataTypeStr=boolean
  xxRollAutopilotSpec_65_operator : Logic  Operator=OR  AllPortsSameDT=off  OutDataTypeStr=boolean
  xxRollAutopilotSpec_66_operator : Logic  AllPortsSameDT=off  OutDataTypeStr=boolean
  xxRollAutopilotSpec_69_operator : Logic  Operator=NOT  AllPortsSameDT=off  OutDataTypeStr=boolean
  xxRollAutopilotSpec_6_operator : cocosimLibs/Implies  SystemSampleTime=-1  Latency=0  AutoFrameSizeCalculation=off
  xxRollAutopilotSpec_70_operator : Logic  AllPortsSameDT=off  OutDataTypeStr=boolean
  xxRollAutopilotSpec_71_operator : Logic  Operator=NOT  AllPortsSameDT=off  OutDataTypeStr=boolean
  xxRollAutopilotSpec_72_operator : Logic  Operator=NOT  AllPortsSameDT=off  OutDataTypeStr=boolean
  xxRollAutopilotSpec_74_operator : Logic  Operator=OR  AllPortsSameDT=off  OutDataTypeStr=boolean
  xxRollAutopilotSpec_75_operator : Logic  AllPortsSameDT=off  OutDataTypeStr=boolean
  xxRollAutopilotSpec_77_operator : cocosimLibs/Implies  SystemSampleTime=-1  Latency=0  AutoFrameSizeCalculation=off
  xxRollAutopilotSpec_78_operator : RelationalOperator  Operator===  OutDataTypeStr=boolean  RndMeth=Simplest
  xxRollAutopilotSpec_78_rhs_2 : Constant  Value=0.0  OutDataTypeStr=double
  xxRollAutopilotSpec_79_operator : RelationalOperator  Operator=>  OutDataTypeStr=boolean  RndMeth=Simplest
  xxRollAutopilotSpec_79_rhs_2 : Constant  Value=-6.0  OutDataTypeStr=double
  xxRollAutopilotSpec_7_operator : Logic  Operator=NOT  AllPortsSameDT=off  OutDataTypeStr=boolean
  xxRollAutopilotSpec_80_operator : RelationalOperator  Operator=<  OutDataTypeStr=boolean  RndMeth=Simplest
  xxRollAutopilotSpec_80_rhs_2 : Constant  Value=6.0  OutDataTypeStr=double
  xxRollAutopilotSpec_81_operator : Logic  AllPortsSameDT=off  OutDataTypeStr=boolean
  xxRollAutopilotSpec_82_operator : cocosimLibs/Implies  SystemSampleTime=-1  Latency=0  AutoFrameSizeCalculation=off
  xxRollAutopilotSpec_83_operator : Logic  Operator=NOT  AllPortsSameDT=off  OutDataTypeStr=boolean
  xxRollAutopilotSpec_85_operator : Logic  Operator=OR  AllPortsSameDT=off  OutDataTypeStr=boolean
  xxRollAutopilotSpec_86_operator : Logic  AllPortsSameDT=off  OutDataTypeStr=boolean
  xxRollAutopilotSpec_87_operator : cocosimLibs/Implies  SystemSampleTime=-1  Latency=0  AutoFrameSizeCalculation=off
  xxRollAutopilotSpec_88_operator : Logic  Operator=NOT  AllPortsSameDT=off  OutDataTypeStr=boolean
  xxRollAutopilotSpec_90_operator : Logic  Operator=OR  AllPortsSameDT=off  OutDataTypeStr=boolean
  xxRollAutopilotSpec_91_operator : Logic  AllPortsSameDT=off  OutDataTypeStr=boolean
  xxRollAutopilotSpec_94_operator : Logic  Operator=NOT  AllPortsSameDT=off  OutDataTypeStr=boolean
  xxRollAutopilotSpec_96_operator : Logic  Operator=NOT  AllPortsSameDT=off  OutDataTypeStr=boolean
  xxRollAutopilotSpec_97_operator : Logic  AllPortsSameDT=off  OutDataTypeStr=boolean
  xxRollAutopilotSpec_98_operator : Logic  AllPortsSameDT=off  OutDataTypeStr=boolean
  xxRollAutopilotSpec_99_operator : cocosimLibs/Implies  SystemSampleTime=-1  Latency=0  AutoFrameSizeCalculation=off
  xxRollAutopilotSpec_9_operator : Logic  Operator=OR  AllPortsSameDT=off  OutDataTypeStr=boolean
  valid : Outport
  wires:
  validator/1 -> valid/1
  PRE_xxRollAutopilotSpec_8/1 -> xxRollAutopilotSpec_9_operator/2
  PRE_xxRollAutopilotSpec_93/1 -> xxRollAutopilotSpec_99_operator/2
  xxRollAutopilotSpec_98_operator/1 -> xxRollAutopilotSpec_99_operator/1
  xxRollAutopilotSpec_94_operator/1 -> xxRollAutopilotSpec_98_operator/2
  xxRollAutopilotSpec_97_operator/1 -> xxRollAutopilotSpec_98_operator/1
  PRE_xxRollAutopilotSpec_95/1 -> xxRollAutopilotSpec_97_operator/2
  xxRollAutopilotSpec_96_operator/1 -> xxRollAutopilotSpec_97_operator/1
  xxRollAutopilotSpec_90_operator/1 -> xxRollAutopilotSpec_91_operator/2
  PRE_xxRollAutopilotSpec_89/1 -> xxRollAutopilotSpec_90_operator/2
  xxRollAutopilotSpec_82_operator/1 -> xxRollAutopilotSpec_87_operator/2
  xxRollAutopilotSpec_86_operator/1 -> xxRollAutopilotSpec_87_operator/1
  xxRollAutopilotSpec_85_operator/1 -> xxRollAutopilotSpec_86_operator/2
  PRE_xxRollAutopilotSpec_84/1 -> xxRollAutopilotSpec_85_operator/2
  xxRollAutopilotSpec_78_operator/1 -> xxRollAutopilotSpec_82_operator/2
  xxRollAutopilotSpec_81_operator/1 -> xxRollAutopilotSpec_82_operator/1
  xxRollAutopilotSpec_79_operator/1 -> xxRollAutopilotSpec_81_operator/2
  xxRollAutopilotSpec_80_operator/1 -> xxRollAutopilotSpec_81_operator/1
  xxRollAutopilotSpec_80_rhs_2/1 -> xxRollAutopilotSpec_80_operator/2
  xxRollAutopilotSpec_79_rhs_2/1 -> xxRollAutopilotSpec_79_operator/2
  xxRollAutopilotSpec_78_rhs_2/1 -> xxRollAutopilotSpec_78_operator/2
  SI_call111/1(SI_Z) -> xxRollAutopilotSpec_77_operator/2
  SI_call11/1(SI_Z) -> xxRollAutopilotSpec_77_operator/1
  xxRollAutopilotSpec_74_operator/1 -> xxRollAutopilotSpec_75_operator/2
  PRE_xxRollAutopilotSpec_73/1 -> xxRollAutopilotSpec_74_operator/2
  xxRollAutopilotSpec_70_operator/1 -> xxRollAutopilotSpec_71_operator/1
  PRE_xxRollAutopilotSpec_68/1 -> xxRollAutopilotSpec_70_operator/2
  xxRollAutopilotSpec_69_operator/1 -> xxRollAutopilotSpec_70_operator/1
  xxRollAutopilotSpec_2_operator/1 -> xxRollAutopilotSpec_6_operator/2
  xxRollAutopilotSpec_5_operator/1 -> xxRollAutopilotSpec_6_operator/1
  xxRollAutopilotSpec_65_operator/1 -> xxRollAutopilotSpec_66_operator/2
  PRE_xxRollAutopilotSpec_64/1 -> xxRollAutopilotSpec_65_operator/2
  xxRollAutopilotSpec_57_operator/1 -> xxRollAutopilotSpec_62_operator/2
  xxRollAutopilotSpec_61_operator/1 -> xxRollAutopilotSpec_62_operator/1
  xxRollAutopilotSpec_60_operator/1 -> xxRollAutopilotSpec_61_operator/2
  PRE_xxRollAutopilotSpec_59/1 -> xxRollAutopilotSpec_60_operator/2
  xxRollAutopilotSpec_4_operator/1 -> xxRollAutopilotSpec_5_operator/1
  xxRollAutopilotSpec_53_operator/1 -> xxRollAutopilotSpec_57_operator/2
  xxRollAutopilotSpec_56_operator/1 -> xxRollAutopilotSpec_57_operator/1
  xxRollAutopilotSpec_54_operator/1 -> xxRollAutopilotSpec_56_operator/2
  xxRollAutopilotSpec_55_operator/1 -> xxRollAutopilotSpec_56_operator/1
  xxRollAutopilotSpec_55_rhs_2/1 -> xxRollAutopilotSpec_55_operator/2
  xxRollAutopilotSpec_54_rhs_2/1 -> xxRollAutopilotSpec_54_operator/2
  xxRollAutopilotSpec_53_rhs_2/1 -> xxRollAutopilotSpec_53_operator/2
  xxRollAutopilotSpec_26_operator/1 -> xxRollAutopilotSpec_50_operator/2
  H_call/1(H_Y) -> xxRollAutopilotSpec_50_operator/1
  xxRollAutopilotSpec_3_operator/1 -> xxRollAutopilotSpec_4_operator/1
  PRE_xxRollAutopilotSpec_42/1 -> xxRollAutopilotSpec_48_operator/2
  xxRollAutopilotSpec_47_operator/1 -> xxRollAutopilotSpec_48_operator/1
  xxRollAutopilotSpec_43_operator/1 -> xxRollAutopilotSpec_47_operator/2
  xxRollAutopilotSpec_46_operator/1 -> xxRollAutopilotSpec_47_operator/1
  PRE_xxRollAutopilotSpec_44/1 -> xxRollAutopilotSpec_46_operator/2
  xxRollAutopilotSpec_45_operator/1 -> xxRollAutopilotSpec_46_operator/1
  xxRollAutopilotSpec_39_operator/1 -> xxRollAutopilotSpec_40_operator/2
  PRE_xxRollAutopilotSpec_38/1 -> xxRollAutopilotSpec_39_operator/2
  xxRollAutopilotSpec_31_operator/1 -> xxRollAutopilotSpec_36_operator/2
  xxRollAutopilotSpec_35_operator/1 -> xxRollAutopilotSpec_36_operator/1
  xxRollAutopilotSpec_34_operator/1 -> xxRollAutopilotSpec_35_operator/2
  PRE_xxRollAutopilotSpec_33/1 -> xxRollAutopilotSpec_34_operator/2
  xxRollAutopilotSpec_27_operator/1 -> xxRollAutopilotSpec_31_operator/2
  xxRollAutopilotSpec_30_operator/1 -> xxRollAutopilotSpec_31_operator/1
  xxRollAutopilotSpec_29_operator/1 -> xxRollAutopilotSpec_30_operator/1
  xxRollAutopilotSpec_28_operator/1 -> xxRollAutopilotSpec_29_operator/1
  SI_call1/1(SI_Z) -> xxRollAutopilotSpec_26_operator/2
  SI_call/1(SI_Z) -> xxRollAutopilotSpec_26_operator/1
  xxRollAutopilotSpec_23_operator/1 -> xxRollAutopilotSpec_24_operator/2
  PRE_xxRollAutopilotSpec_22/1 -> xxRollAutopilotSpec_23_operator/2
  xxRollAutopilotSpec_19_operator/1 -> xxRollAutopilotSpec_20_operator/1
  PRE_xxRollAutopilotSpec_17/1 -> xxRollAutopilotSpec_19_operator/2
  xxRollAutopilotSpec_18_operator/1 -> xxRollAutopilotSpec_19_operator/1
  xxRollAutopilotSpec_181_operator/1 -> xxRollAutopilotSpec_182_operator/1
  xxRollAutopilotSpec_178_operator/1 -> xxRollAutopilotSpec_180_operator/2
  xxRollAutopilotSpec_179_operator/1 -> xxRollAutopilotSpec_180_operator/1
  xxRollAutopilotSpec_179_rhs_2/1 -> xxRollAutopilotSpec_179_operator/2
  xxRollAutopilotSpec_178_rhs_2/1 -> xxRollAutopilotSpec_178_operator/2
  xxRollAutopilotSpec_175_operator/1 -> xxRollAutopilotSpec_177_operator/2
  xxRollAutopilotSpec_176_operator/1 -> xxRollAutopilotSpec_177_operator/1
  xxRollAutopilotSpec_176_rhs_2/1 -> xxRollAutopilotSpec_176_operator/2
  xxRollAutopilotSpec_175_rhs_2/1 -> xxRollAutopilotSpec_175_operator/2
  xxRollAutopilotSpec_174_rhs_2/1 -> xxRollAutopilotSpec_174_operator/2
  xxRollAutopilotSpec_173_rhs_2/1 -> xxRollAutopilotSpec_173_operator/2
  xxRollAutopilotSpec_169_rhs_2/1 -> xxRollAutopilotSpec_169_operator/2
  xxRollAutopilotSpec_167_rhs_2/1 -> xxRollAutopilotSpec_167_operator/2
  xxRollAutopilotSpec_160_rhs_2/1 -> xxRollAutopilotSpec_160_operator/2
  xxRollAutopilotSpec_14_operator/1 -> xxRollAutopilotSpec_15_operator/2
  xxRollAutopilotSpec_155_operator/1 -> xxRollAutopilotSpec_159_operator/2
  xxRollAutopilotSpec_158_operator/1 -> xxRollAutopilotSpec_159_operator/1
  xxRollAutopilotSpec_156_operator/1 -> xxRollAutopilotSpec_158_operator/2
  xxRollAutopilotSpec_157_operator/1 -> xxRollAutopilotSpec_158_operator/1
  xxRollAutopilotSpec_157_rhs_2/1 -> xxRollAutopilotSpec_157_operator/2
  xxRollAutopilotSpec_156_rhs_2/1 -> xxRollAutopilotSpec_156_operator/2
  xxRollAutopilotSpec_153_operator/1 -> xxRollAutopilotSpec_155_operator/2
  xxRollAutopilotSpec_154_operator/1 -> xxRollAutopilotSpec_155_operator/1
  xxRollAutopilotSpec_154_rhs_2/1 -> xxRollAutopilotSpec_154_operator/2
  xxRollAutopilotSpec_153_rhs_2/1 -> xxRollAutopilotSpec_153_operator/2
  xxRollAutopilotSpec_127_operator/1 -> xxRollAutopilotSpec_150_operator/2
  H_call11/1(H_Y) -> xxRollAutopilotSpec_150_operator/1
  PRE_xxRollAutopilotSpec_13/1 -> xxRollAutopilotSpec_14_operator/2
  PRE_xxRollAutopilotSpec_142/1 -> xxRollAutopilotSpec_148_operator/2
  xxRollAutopilotSpec_147_operator/1 -> xxRollAutopilotSpec_148_operator/1
  xxRollAutopilotSpec_143_operator/1 -> xxRollAutopilotSpec_147_operator/2
  xxRollAutopilotSpec_146_operator/1 -> xxRollAutopilotSpec_147_operator/1
  PRE_xxRollAutopilotSpec_144/1 -> xxRollAutopilotSpec_146_operator/2
  xxRollAutopilotSpec_145_operator/1 -> xxRollAutopilotSpec_146_operator/1
  xxRollAutopilotSpec_139_operator/1 -> xxRollAutopilotSpec_140_operator/2
  PRE_xxRollAutopilotSpec_138/1 -> xxRollAutopilotSpec_139_operator/2
  xxRollAutopilotSpec_131_operator/1 -> xxRollAutopilotSpec_136_operator/2
  xxRollAutopilotSpec_135_operator/1 -> xxRollAutopilotSpec_136_operator/1
  xxRollAutopilotSpec_134_operator/1 -> xxRollAutopilotSpec_135_operator/2
  PRE_xxRollAutopilotSpec_133/1 -> xxRollAutopilotSpec_134_operator/2
  xxRollAutopilotSpec_129_operator/1 -> xxRollAutopilotSpec_131_operator/2
  xxRollAutopilotSpec_130_operator/1 -> xxRollAutopilotSpec_131_operator/1
  xxRollAutopilotSpec_130_rhs_2/1 -> xxRollAutopilotSpec_130_operator/2
  xxRollAutopilotSpec_128_operator/1 -> xxRollAutopilotSpec_129_operator/2
  xxRollAutopilotSpec_128_rhs_1/1 -> xxRollAutopilotSpec_128_operator/1
  SI_call11111/1(SI_Z) -> xxRollAutopilotSpec_127_operator/2
  SI_call1111/1(SI_Z) -> xxRollAutopilotSpec_127_operator/1
  xxRollAutopilotSpec_124_operator/1 -> xxRollAutopilotSpec_125_operator/2
  PRE_xxRollAutopilotSpec_123/1 -> xxRollAutopilotSpec_124_operator/2
  xxRollAutopilotSpec_120_operator/1 -> xxRollAutopilotSpec_121_operator/1
  PRE_xxRollAutopilotSpec_118/1 -> xxRollAutopilotSpec_120_operator/2
  xxRollAutopilotSpec_119_operator/1 -> xxRollAutopilotSpec_120_operator/1
  xxRollAutopilotSpec_6_operator/1 -> xxRollAutopilotSpec_11_operator/2
  xxRollAutopilotSpec_10_operator/1 -> xxRollAutopilotSpec_11_operator/1
  xxRollAutopilotSpec_115_operator/1 -> xxRollAutopilotSpec_116_operator/2
  PRE_xxRollAutopilotSpec_114/1 -> xxRollAutopilotSpec_115_operator/2
  xxRollAutopilotSpec_107_operator/1 -> xxRollAutopilotSpec_112_operator/2
  xxRollAutopilotSpec_111_operator/1 -> xxRollAutopilotSpec_112_operator/1
  xxRollAutopilotSpec_110_operator/1 -> xxRollAutopilotSpec_111_operator/2
  PRE_xxRollAutopilotSpec_109/1 -> xxRollAutopilotSpec_110_operator/2
  xxRollAutopilotSpec_9_operator/1 -> xxRollAutopilotSpec_10_operator/2
  xxRollAutopilotSpec_105_operator/1 -> xxRollAutopilotSpec_107_operator/2
  xxRollAutopilotSpec_106_operator/1 -> xxRollAutopilotSpec_107_operator/1
  xxRollAutopilotSpec_106_rhs_2/1 -> xxRollAutopilotSpec_106_operator/2
  xxRollAutopilotSpec_104_operator/1 -> xxRollAutopilotSpec_105_operator/2
  xxRollAutopilotSpec_104_rhs_1/1 -> xxRollAutopilotSpec_104_operator/1
  xxRollAutopilotSpec_77_operator/1 -> xxRollAutopilotSpec_101_operator/2
  H_call1/1(H_Y) -> xxRollAutopilotSpec_101_operator/1
  hdg_hold_mode/1(mode) -> validator/8
  roll_hold_mode/1(mode) -> validator/7
  AP-007/1(guarantee) -> validator/6
  AP-003A/1(guarantee) -> validator/5
  AP-003B/1(guarantee) -> validator/4
  AP-003C/1(guarantee) -> validator/3
  AP-003D/1(guarantee) -> validator/2
  AP-001/1(guarantee) -> validator/1
  spec621_rhs_2/1 -> spec621_operator/2
  branch_8_IF/1 -> spec621_operator/1
  xxRollAutopilotSpec_152_operator/1 -> spec252_operator/2
  xxRollAutopilotSpec_159_operator/1 -> spec252_operator/1
  RollAutopilotSpec_hdg_hold_mode_cmd/1 -> spec223_operator/2
  xxRollAutopilotSpec_160_operator/1 -> spec206_operator/2
  xxRollAutopilotSpec_161_operator/1 -> spec206_operator/1
  spec211_operator/1 -> roll_hold_mode_require_cond/1
  roll_hold_mode_require_cond/1 -> roll_hold_mode_require/1(In1)
  spec216_operator/1 -> roll_hold_mode_ensure_cond/1
  roll_hold_mode_ensure_cond/1 -> roll_hold_mode_ensure/1(In1)
  roll_hold_mode_ensure/1(ensure) -> roll_hold_mode/2(ensure)
  roll_hold_mode_require/1(require) -> roll_hold_mode/1(require)
  branch_15_IF/1 -> [RollAutopilotSpec_pre_roll_angle]
  branch_16_IF/1 -> [RollAutopilotSpec_pre_Ca]
  hdg_hold_mode_require_cond/1 -> hdg_hold_mode_require/1(In1)
  spec223_operator/1 -> hdg_hold_mode_ensure_cond/1
  hdg_hold_mode_ensure_cond/1 -> hdg_hold_mode_ensure/1(In1)
  hdg_hold_mode_ensure/1(ensure) -> hdg_hold_mode/2(ensure)
  hdg_hold_mode_require/1(require) -> hdg_hold_mode/1(require)
  xxRollAutopilotSpec_170_operator/1 -> branch_9_IF/3
  xxRollAutopilotSpec_168_operator/1 -> branch_8_IF/3
  xxRollAutopilotSpec_167_operator/1 -> branch_8_IF/2
  PRE_xxRollAutopilotSpec_184/1 -> branch_16_IF/3
  xxRollAutopilotSpec_185_rhs1/1 -> branch_16_IF/1
  PRE_xxRollAutopilotSpec_187/1 -> branch_15_IF/3
  xxRollAutopilotSpec_186_rhs/1 -> branch_15_IF/1
  xxRollAutopilotSpec_150_operator/1 -> branch_14_IF/3
  Arrow_xxRollAutopilotSpec_162_ni_7/1 -> branch_14_IF/2
  xxRollAutopilotSpec_151_rhs1/1 -> branch_14_IF/1
  xxRollAutopilotSpec_172_rhs/1 -> branch_13_IF/3
  xxRollAutopilotSpec_171_rhs/1 -> branch_13_IF/1
  xxRollAutopilotSpec_101_operator/1 -> branch_12_IF/3
  Arrow_xxRollAutopilotSpec_163_ni_9/1 -> branch_12_IF/2
  xxRollAutopilotSpec_102_rhs1/1 -> branch_12_IF/1
  xxRollAutopilotSpec_50_operator/1 -> branch_11_IF/3
  Arrow_xxRollAutopilotSpec_164_ni_12/1 -> branch_11_IF/2
  xxRollAutopilotSpec_51_rhs1/1 -> branch_11_IF/1
  xxRollAutopilotSpec_166_rhs/1 -> branch_10_IF/3
  Arrow_xxRollAutopilotSpec_165_ni_16/1 -> branch_10_IF/2
  xxRollAutopilotSpec_166_rhs1/1 -> branch_10_IF/1
  xxRollAutopilotSpec_136_operator/1 -> SI_call11111111/2(SI_Y)
  xxRollAutopilotSpec_140_operator/1 -> SI_call11111111/1(SI_X)
  xxRollAutopilotSpec_36_operator/1 -> SI_call1111111/2(SI_Y)
  xxRollAutopilotSpec_40_operator/1 -> SI_call1111111/1(SI_X)
  xxRollAutopilotSpec_87_operator/1 -> SI_call111111/2(SI_Y)
  xxRollAutopilotSpec_91_operator/1 -> SI_call111111/1(SI_X)
  xxRollAutopilotSpec_112_operator/1 -> SI_call11111/2(SI_Y)
  xxRollAutopilotSpec_116_operator/1 -> SI_call11111/1(SI_X)
  xxRollAutopilotSpec_121_operator/1 -> SI_call1111/2(SI_Y)
  xxRollAutopilotSpec_125_operator/1 -> SI_call1111/1(SI_X)
  xxRollAutopilotSpec_62_operator/1 -> SI_call111/2(SI_Y)
  xxRollAutopilotSpec_66_operator/1 -> SI_call111/1(SI_X)
  xxRollAutopilotSpec_71_operator/1 -> SI_call11/2(SI_Y)
  xxRollAutopilotSpec_75_operator/1 -> SI_call11/1(SI_X)
  xxRollAutopilotSpec_11_operator/1 -> SI_call1/2(SI_Y)
  xxRollAutopilotSpec_15_operator/1 -> SI_call1/1(SI_X)
  xxRollAutopilotSpec_20_operator/1 -> SI_call/2(SI_Y)
  xxRollAutopilotSpec_24_operator/1 -> SI_call/1(SI_X)
  SI_call111111/1(SI_Z) -> PRE_xxRollAutopilotSpec_93/1
  xxRollAutopilotSpec_88_operator/1 -> PRE_xxRollAutopilotSpec_89/1
  xxRollAutopilotSpec_83_operator/1 -> PRE_xxRollAutopilotSpec_84/1
  xxRollAutopilotSpec_7_operator/1 -> PRE_xxRollAutopilotSpec_8/1
  xxRollAutopilotSpec_72_operator/1 -> PRE_xxRollAutopilotSpec_73/1
  xxRollAutopilotSpec_63_operator/1 -> PRE_xxRollAutopilotSpec_64/1
  xxRollAutopilotSpec_58_operator/1 -> PRE_xxRollAutopilotSpec_59/1
  SI_call1111111/1(SI_Z) -> PRE_xxRollAutopilotSpec_42/1
  xxRollAutopilotSpec_37_operator/1 -> PRE_xxRollAutopilotSpec_38/1
  xxRollAutopilotSpec_32_operator/1 -> PRE_xxRollAutopilotSpec_33/1
  xxRollAutopilotSpec_21_operator/1 -> PRE_xxRollAutopilotSpec_22/1
  Ca_operator/1 -> PRE_xxRollAutopilotSpec_184/1
  SI_call11111111/1(SI_Z) -> PRE_xxRollAutopilotSpec_142/1
  xxRollAutopilotSpec_137_operator/1 -> PRE_xxRollAutopilotSpec_138/1
  xxRollAutopilotSpec_132_operator/1 -> PRE_xxRollAutopilotSpec_133/1
  xxRollAutopilotSpec_12_operator/1 -> PRE_xxRollAutopilotSpec_13/1
  xxRollAutopilotSpec_122_operator/1 -> PRE_xxRollAutopilotSpec_123/1
  xxRollAutopilotSpec_113_operator/1 -> PRE_xxRollAutopilotSpec_114/1
  xxRollAutopilotSpec_108_operator/1 -> PRE_xxRollAutopilotSpec_109/1
  xxRollAutopilotSpec_148_operator/1 -> H_call11/1(H_X)
  xxRollAutopilotSpec_99_operator/1 -> H_call1/1(H_X)
  xxRollAutopilotSpec_48_operator/1 -> H_call/1(H_X)
  xxRollAutopilotSpec_177_operator/1 -> Cd_operator/2
  xxRollAutopilotSpec_180_operator/1 -> Cd_operator/1
  Cc_rhs_2/1 -> Cc_operator/2
  xxRollAutopilotSpec_173_operator/1 -> Cb_operator/2
  xxRollAutopilotSpec_174_operator/1 -> Cb_operator/1
  xxRollAutopilotSpec_182_operator/1 -> Ca_operator/1
  xxRollAutopilotSpec_183_ni_3_init/1 -> Arrow_xxRollAutopilotSpec_183_ni_3/1
  xxRollAutopilotSpec_165_ni_16_init/1 -> Arrow_xxRollAutopilotSpec_165_ni_16/1
  xxRollAutopilotSpec_164_ni_12_init/1 -> Arrow_xxRollAutopilotSpec_164_ni_12/1
  xxRollAutopilotSpec_163_ni_9_init/1 -> Arrow_xxRollAutopilotSpec_163_ni_9/1
  xxRollAutopilotSpec_162_ni_7_init/1 -> Arrow_xxRollAutopilotSpec_162_ni_7/1
  spec621_operator/1 -> AP-007/1(In1)
  spec252_operator/1 -> AP-003D/1(In1)
  branch_14_IF/1 -> AP-003C/1(In1)
  branch_12_IF/1 -> AP-003B/1(In1)
  branch_11_IF/1 -> AP-003A/1(In1)
  spec206_operator/1 -> AP-001/1(In1)
  RollAutopilotSpec_HDGmode/1 -> no_other_lateral_mode_operator/1, hdg_hold_mode_require_cond/1
  roll_hold_operator/1 -> xxRollAutopilotSpec_15_operator/1, xxRollAutopilotSpec_10_operator/1, xxRollAutopilotSpec_18_operator/1, xxRollAutopilotSpec_24_operator/1, xxRollAutopilotSpec_45_operator/1, xxRollAutopilotSpec_66_operator/1, xxRollAutopilotSpec_61_operator/1, xxRollAutopilotSpec_69_operator/1, xxRollAutopilotSpec_75_operator/1, xxRollAutopilotSpec_96_operator/1, xxRollAutopilotSpec_116_operator/1, xxRollAutopilotSpec_111_operator/1, xxRollAutopilotSpec_119_operator/1, xxRollAutopilotSpec_125_operator/1, xxRollAutopilotSpec_145_operator/1, xxRollAutopilotSpec_91_operator/1, xxRollAutopilotSpec_86_operator/1, PRE_xxRollAutopilotSpec_144/1, PRE_xxRollAutopilotSpec_118/1, PRE_xxRollAutopilotSpec_17/1, PRE_xxRollAutopilotSpec_44/1, PRE_xxRollAutopilotSpec_68/1, xxRollAutopilotSpec_113_operator/1, xxRollAutopilotSpec_108_operator/1, xxRollAutopilotSpec_122_operator/1, xxRollAutopilotSpec_12_operator/1, xxRollAutopilotSpec_132_operator/1, xxRollAutopilotSpec_137_operator/1, xxRollAutopilotSpec_135_operator/1, xxRollAutopilotSpec_140_operator/1, xxRollAutopilotSpec_21_operator/1, xxRollAutopilotSpec_32_operator/1, xxRollAutopilotSpec_37_operator/1, xxRollAutopilotSpec_35_operator/1, xxRollAutopilotSpec_40_operator/1, xxRollAutopilotSpec_58_operator/1, xxRollAutopilotSpec_63_operator/1, xxRollAutopilotSpec_72_operator/1, xxRollAutopilotSpec_7_operator/1, xxRollAutopilotSpec_83_operator/1, xxRollAutopilotSpec_88_operator/1, PRE_xxRollAutopilotSpec_95/1
  Cd_operator/1 -> xxRollAutopilotSpec_29_operator/2, xxRollAutopilotSpec_182_operator/2, xxRollAutopilotSpec_4_operator/2
  Cc_operator/1 -> xxRollAutopilotSpec_28_operator/2, xxRollAutopilotSpec_181_operator/2, xxRollAutopilotSpec_3_operator/2
  Cb_operator/1 -> xxRollAutopilotSpec_28_operator/1, xxRollAutopilotSpec_181_operator/1, xxRollAutopilotSpec_3_operator/1
  Arrow_xxRollAutopilotSpec_183_ni_3/1 -> branch_16_IF/2, branch_15_IF/2
  RollAutopilotSpec_roll_hold_reference/1 -> xxRollAutopilotSpec_152_operator/1, spec216_operator/2, xxRollAutopilotSpec_27_operator/1, xxRollAutopilotSpec_129_operator/1, xxRollAutopilotSpec_78_operator/1, xxRollAutopilotSpec_105_operator/1, xxRollAutopilotSpec_53_operator/1, xxRollAutopilotSpec_2_operator/1
  RollAutopilotSpec_roll_cmd/1 -> spec223_operator/1, spec216_operator/1
  RollAutopilotSpec_TurnKnob/1 -> xxRollAutopilotSpec_176_operator/1, xxRollAutopilotSpec_175_operator/1, xxRollAutopilotSpec_178_operator/1, xxRollAutopilotSpec_179_operator/1, xxRollAutopilotSpec_153_operator/1, xxRollAutopilotSpec_152_operator/2, xxRollAutopilotSpec_154_operator/1, xxRollAutopilotSpec_156_operator/1, xxRollAutopilotSpec_157_operator/1
  branch_13_IF/1 -> xxRollAutopilotSpec_128_operator/2, xxRollAutopilotSpec_104_operator/2
  branch_10_IF/1 -> xxRollAutopilotSpec_23_operator/1, xxRollAutopilotSpec_14_operator/1, xxRollAutopilotSpec_43_operator/1, xxRollAutopilotSpec_9_operator/1, xxRollAutopilotSpec_65_operator/1, xxRollAutopilotSpec_60_operator/1, xxRollAutopilotSpec_74_operator/1, xxRollAutopilotSpec_94_operator/1, xxRollAutopilotSpec_115_operator/1, xxRollAutopilotSpec_110_operator/1, xxRollAutopilotSpec_124_operator/1, xxRollAutopilotSpec_143_operator/1, xxRollAutopilotSpec_90_operator/1, xxRollAutopilotSpec_85_operator/1, xxRollAutopilotSpec_139_operator/1, xxRollAutopilotSpec_134_operator/1, xxRollAutopilotSpec_34_operator/1, xxRollAutopilotSpec_39_operator/1
  xxRollAutopilotSpec_169_operator/1 -> branch_9_IF/2, branch_13_IF/2
  branch_9_IF/1 -> xxRollAutopilotSpec_130_operator/1, xxRollAutopilotSpec_106_operator/1, Cc_operator/1
  RollAutopilotSpec_roll_angle/1 -> xxRollAutopilotSpec_170_operator/1, xxRollAutopilotSpec_169_operator/1, xxRollAutopilotSpec_2_operator/2, xxRollAutopilotSpec_173_operator/1, xxRollAutopilotSpec_174_operator/1, xxRollAutopilotSpec_55_operator/1, xxRollAutopilotSpec_54_operator/1, xxRollAutopilotSpec_80_operator/1, xxRollAutopilotSpec_79_operator/1, xxRollAutopilotSpec_27_operator/2, PRE_xxRollAutopilotSpec_187/1, branch_9_IF/1
  RollAutopilotSpec_autopilot_engaged/1 -> xxRollAutopilotSpec_161_operator/1, spec211_operator/2, roll_hold_operator/2
  no_other_lateral_mode_operator/1 -> spec211_operator/1, roll_hold_operator/1
  RollAutopilotSpec_roll_actuator_command/1 -> xxRollAutopilotSpec_168_operator/1, xxRollAutopilotSpec_167_operator/1, xxRollAutopilotSpec_160_operator/1, branch_8_IF/1
